simulink model "SimulinkModel"  (R2023b)
settings: Solver=VariableStepAuto  StartTime=0.0  StopTime=10.0  RelTol=1e-3
libraries: simulink x20, simulink_extras x7
settings Model: Creator=oykusucuoglu  LastModifiedBy=oykusucuoglu
settings OptimizationCC: ReuseModelBlockBuffer=off

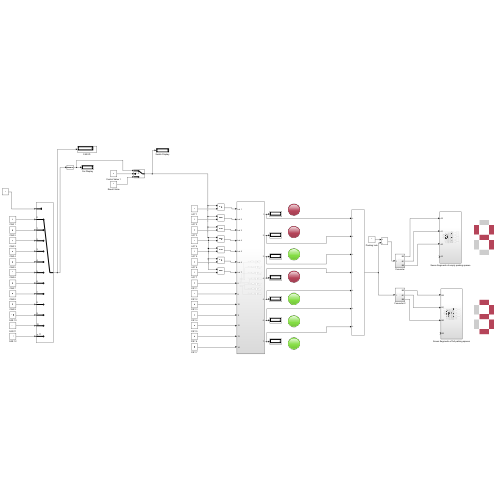
[thumbnail: Simulink's stored preview of the top-level diagram]
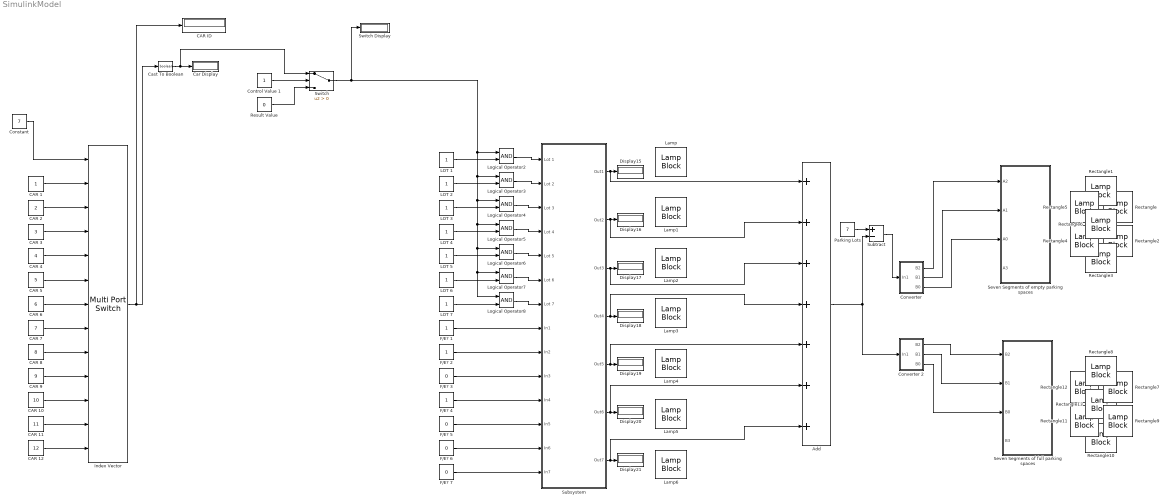
== system SimulinkModel ==
  Add : Sum  Inputs=+++++++
  CAR 1 : Constant
  CAR 10 : Constant  Value=10
  CAR 11 : Constant  Value=11
  CAR 12 : Constant  Value=12
  CAR 2 : Constant  Value=2
  CAR 3 : Constant  Value=3
  CAR 4 : Constant  Value=4
  CAR 5 : Constant  Value=5
  CAR 6 : Constant  Value=6
  CAR 7 : Constant  Value=7
  CAR 8 : Constant  Value=8
  CAR 9 : Constant  Value=9
  "CAR ID " : Display
  Car Display : Display
  Cast To Boolean : DataTypeConversion  OutDataTypeStr=boolean  SaturateOnIntegerOverflow=off  RndMeth=Floor
  Constant : Constant  Value=7
  Control Value 1 : Constant
  Converter : Subsystem
  Converter 2 : Subsystem
  Display{15..21} (7 alike) : Display
  F/E? 1 : Constant
  F/E? 2 : Constant
  F/E? 3 : Constant  Value=0
  F/E? 4 : Constant
  F/E? 5 : Constant  Value=0
  "F/E? 6 " : Constant  Value=0
  F/E? 7 : Constant  Value=0
  Index Vector : MultiPortSwitch  DataPortOrder=Zero-based contiguous  Inputs=12  zeroidx=on  SaturateOnIntegerOverflow=off  InputSameDT=off
  LOT {1..7} (7 alike) : Constant
  Lamp{,1..6} (7 alike) : LampBlock  LabelPosition=Hide
  Logical Operator{2..8} (7 alike) : Logic  AllPortsSameDT=off  OutDataTypeStr=boolean
  Parking Lots : Constant  Value=7
  Rectangle{,1..13} (14 alike) : LampBlock  LabelPosition=Hide  Icon=Rectangle
  Result Value : Constant  Value=0
  Seven Segments of empty parking spaces : Subsystem
  Seven Segments of full parking spaces : Subsystem
  Subsystem : Subsystem
  Subtract : Sum  Inputs=+-
  Switch : Switch  Criteria=u2 > Threshold  SaturateOnIntegerOverflow=off  InputSameDT=off
  Switch Display : Display
  wires:
  CAR 5/1 -> Index Vector/6
  CAR 11/1 -> Index Vector/12
  CAR 3/1 -> Index Vector/4
  CAR 2/1 -> Index Vector/3
  CAR 7/1 -> Index Vector/8
  CAR 10/1 -> Index Vector/11
  CAR 1/1 -> Index Vector/2
  Index Vector/1 -> "CAR ID "/1, Cast To Boolean/1
  CAR 4/1 -> Index Vector/5
  CAR 8/1 -> Index Vector/9
  CAR 6/1 -> Index Vector/7
  Constant/1 -> Index Vector/1
  CAR 12/1 -> Index Vector/13
  CAR 9/1 -> Index Vector/10
  Add/1 -> Converter 2/1(In1), Subtract/2
  Result Value/1 -> Switch/3
  Control Value 1/1 -> Switch/2
  Subsystem/2(Out2) -> Add/2, Display16/1
  Subsystem/3(Out3) -> Add/3, Display17/1
  Subsystem/4(Out4) -> Add/4, Display18/1
  Subsystem/5(Out5) -> Add/5, Display19/1
  Subsystem/6(Out6) -> Add/6, Display20/1
  Subsystem/7(Out7) -> Add/7, Display21/1
  Subsystem/1(Out1) -> Add/1, Display15/1
  Cast To Boolean/1 -> Switch/1, Car Display/1
  Parking Lots/1 -> Subtract/1
  "F/E? 6 "/1 -> Subsystem/13(In6)
  F/E? 4/1 -> Subsystem/11(In4)
  F/E? 7/1 -> Subsystem/14(In7)
  F/E? 1/1 -> Subsystem/8(In1)
  F/E? 5/1 -> Subsystem/12(In5)
  F/E? 3/1 -> Subsystem/10(In3)
  F/E? 2/1 -> Subsystem/9(In2)
  LOT 1/1 -> Logical Operator2/2
  LOT 2/1 -> Logical Operator3/2
  LOT 3/1 -> Logical Operator4/2
  Switch/1 -> Logical Operator8/1, Logical Operator7/1, Logical Operator6/1, Logical Operator5/1, Logical Operator4/1, Logical Operator3/1, Logical Operator2/1, Switch Display/1
  LOT 4/1 -> Logical Operator5/2
  LOT 5/1 -> Logical Operator6/2
  LOT 6/1 -> Logical Operator7/2
  LOT 7/1 -> Logical Operator8/2
  Logical Operator2/1 -> Subsystem/1(Lot 1)
  Logical Operator3/1 -> Subsystem/2(Lot 2)
  Logical Operator4/1 -> Subsystem/3(Lot 3)
  Logical Operator5/1 -> Subsystem/4(Lot 4)
  Logical Operator6/1 -> Subsystem/5(Lot 5)
  Logical Operator7/1 -> Subsystem/6(Lot 6)
  Logical Operator8/1 -> Subsystem/7(Lot 7)
  Subtract/1 -> Converter/1(In1)
  Converter/1(B2) -> Seven Segments of empty parking spaces/1(A2)
  Converter/2(B1) -> Seven Segments of empty parking spaces/2(A1)
  Converter/3(B0) -> Seven Segments of empty parking spaces/3(A0)
  Converter 2/1(B2) -> Seven Segments of full parking spaces/1(B2)
  Converter 2/2(B1) -> Seven Segments of full parking spaces/2(B1)
  Converter 2/3(B0) -> Seven Segments of full parking spaces/3(B0)

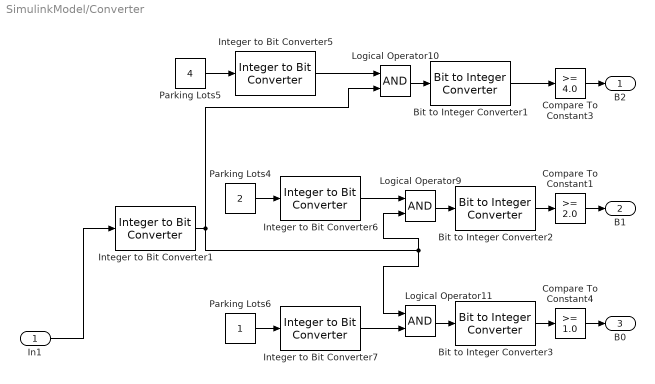
== system SimulinkModel/Converter ==
  In1 : Inport
  Bit to Integer Converter1 : simulink/Logic and Bit Operations/Bit to Integer Converter  nbits=3  bitOrder=MSB first  signedOutputValues=Unsigned  outDtype=Inherit via internal rule  outDtypeSigned=Inherit via internal rule
  Bit to Integer Converter2 : simulink/Logic and Bit Operations/Bit to Integer Converter  nbits=3  bitOrder=MSB first  signedOutputValues=Unsigned  outDtype=Inherit via internal rule  outDtypeSigned=Inherit via internal rule
  Bit to Integer Converter3 : simulink/Logic and Bit Operations/Bit to Integer Converter  nbits=3  bitOrder=MSB first  signedOutputValues=Unsigned  outDtype=Inherit via internal rule  outDtypeSigned=Inherit via internal rule
  Compare To Constant1 : simulink/Logic and Bit Operations/Compare To Constant  relop=>=  const=2.0  OutDataTypeStr=boolean
  Compare To Constant3 : simulink/Logic and Bit Operations/Compare To Constant  relop=>=  const=4.0  OutDataTypeStr=boolean
  Compare To Constant4 : simulink/Logic and Bit Operations/Compare To Constant  relop=>=  const=1.0  OutDataTypeStr=boolean
  Integer to Bit Converter{1,5..7} (4 alike) : simulink/Logic and Bit Operations/Integer to Bit Converter  nbits=3  signedInputValues=Unsigned  bitOrder=MSB first  outDtype=Inherit via internal rule
  Logical Operator10 : Logic  AllPortsSameDT=off  OutDataTypeStr=boolean
  Logical Operator11 : Logic  AllPortsSameDT=off  OutDataTypeStr=boolean
  Logical Operator9 : Logic  AllPortsSameDT=off  OutDataTypeStr=boolean
  Parking Lots4 : Constant  Value=2
  Parking Lots5 : Constant  Value=4
  Parking Lots6 : Constant
  B2 : Outport
  B1 : Outport  Port=2
  B0 : Outport  Port=3
  wires:
  Bit to Integer Converter2/1 -> Compare To Constant1/1
  Integer to Bit Converter1/1 -> Logical Operator10/2, Logical Operator11/1, Logical Operator9/2
  Parking Lots5/1 -> Integer to Bit Converter5/1
  Logical Operator9/1 -> Bit to Integer Converter2/1
  Logical Operator10/1 -> Bit to Integer Converter1/1
  Bit to Integer Converter1/1 -> Compare To Constant3/1
  Integer to Bit Converter7/1 -> Logical Operator11/2
  Integer to Bit Converter5/1 -> Logical Operator10/1
  Parking Lots4/1 -> Integer to Bit Converter6/1
  In1/1 -> Integer to Bit Converter1/1
  Integer to Bit Converter6/1 -> Logical Operator9/1
  Logical Operator11/1 -> Bit to Integer Converter3/1
  Parking Lots6/1 -> Integer to Bit Converter7/1
  Bit to Integer Converter3/1 -> Compare To Constant4/1
  Compare To Constant4/1 -> B0/1
  Compare To Constant1/1 -> B1/1
  Compare To Constant3/1 -> B2/1

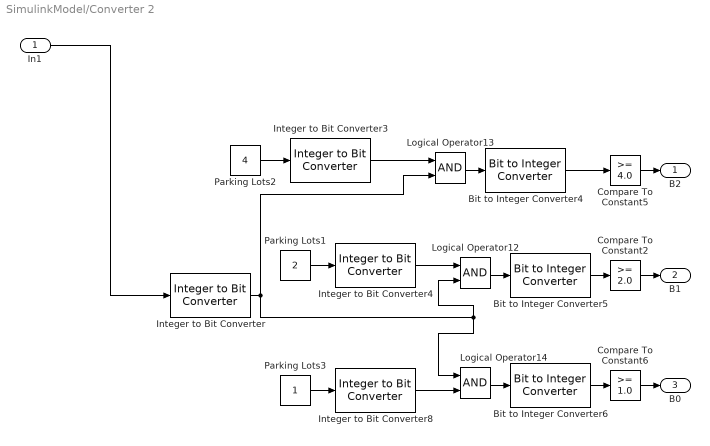
== system SimulinkModel/Converter 2 ==
  In1 : Inport
  Bit to Integer Converter4 : simulink/Logic and Bit Operations/Bit to Integer Converter  nbits=3  bitOrder=MSB first  signedOutputValues=Unsigned  outDtype=Inherit via internal rule  outDtypeSigned=Inherit via internal rule
  Bit to Integer Converter5 : simulink/Logic and Bit Operations/Bit to Integer Converter  nbits=3  bitOrder=MSB first  signedOutputValues=Unsigned  outDtype=Inherit via internal rule  outDtypeSigned=Inherit via internal rule
  Bit to Integer Converter6 : simulink/Logic and Bit Operations/Bit to Integer Converter  nbits=3  bitOrder=MSB first  signedOutputValues=Unsigned  outDtype=Inherit via internal rule  outDtypeSigned=Inherit via internal rule
  Compare To Constant2 : simulink/Logic and Bit Operations/Compare To Constant  relop=>=  const=2.0  OutDataTypeStr=boolean
  Compare To Constant5 : simulink/Logic and Bit Operations/Compare To Constant  relop=>=  const=4.0  OutDataTypeStr=boolean
  Compare To Constant6 : simulink/Logic and Bit Operations/Compare To Constant  relop=>=  const=1.0  OutDataTypeStr=boolean
  Integer to Bit Converter{,3..4,8} (4 alike) : simulink/Logic and Bit Operations/Integer to Bit Converter  nbits=3  signedInputValues=Unsigned  bitOrder=MSB first  outDtype=Inherit via internal rule
  Logical Operator12 : Logic  AllPortsSameDT=off  OutDataTypeStr=boolean
  Logical Operator13 : Logic  AllPortsSameDT=off  OutDataTypeStr=boolean
  Logical Operator14 : Logic  AllPortsSameDT=off  OutDataTypeStr=boolean
  Parking Lots1 : Constant  Value=2
  Parking Lots2 : Constant  Value=4
  Parking Lots3 : Constant
  B2 : Outport
  B1 : Outport  Port=2
  B0 : Outport  Port=3
  wires:
  Compare To Constant2/1 -> B1/1
  Logical Operator12/1 -> Bit to Integer Converter5/1
  Parking Lots2/1 -> Integer to Bit Converter3/1
  Integer to Bit Converter/1 -> Logical Operator13/2, Logical Operator14/1, Logical Operator12/2
  Parking Lots1/1 -> Integer to Bit Converter4/1
  Compare To Constant5/1 -> B2/1
  Logical Operator13/1 -> Bit to Integer Converter4/1
  Bit to Integer Converter4/1 -> Compare To Constant5/1
  Bit to Integer Converter5/1 -> Compare To Constant2/1
  Integer to Bit Converter3/1 -> Logical Operator13/1
  Bit to Integer Converter6/1 -> Compare To Constant6/1
  Logical Operator14/1 -> Bit to Integer Converter6/1
  Integer to Bit Converter8/1 -> Logical Operator14/2
  Integer to Bit Converter4/1 -> Logical Operator12/1
  Parking Lots3/1 -> Integer to Bit Converter8/1
  In1/1 -> Integer to Bit Converter/1
  Compare To Constant6/1 -> B0/1

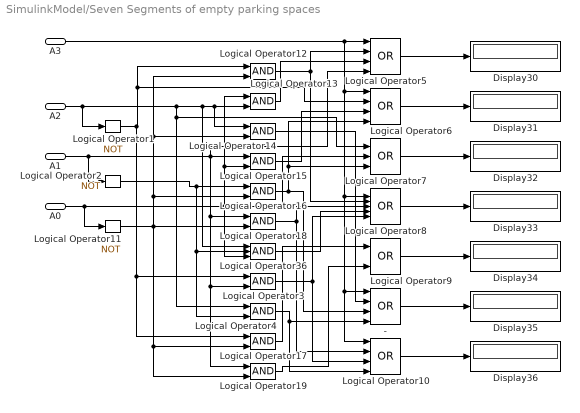
== system SimulinkModel/Seven Segments of empty parking spaces ==
  A2 : Inport
  A1 : Inport  Port=2
  A0 : Inport  Port=3
  A3 : Inport  Port=4
  "   -" : Logic  Operator=OR  Inputs=4  AllPortsSameDT=off  OutDataTypeStr=boolean
  Display{30..36} (7 alike) : Display
  Logical Operator1 : Logic  Operator=NOT  AllPortsSameDT=off  OutDataTypeStr=boolean
  Logical Operator10 : Logic  Operator=OR  Inputs=4  AllPortsSameDT=off  OutDataTypeStr=boolean
  Logical Operator11 : Logic  Operator=NOT  AllPortsSameDT=off  OutDataTypeStr=boolean
  Logical Operator{3..4,12..19} (10 alike) : Logic  AllPortsSameDT=off  OutDataTypeStr=boolean
  Logical Operator2 : Logic  Operator=NOT  AllPortsSameDT=off  OutDataTypeStr=boolean
  Logical Operator36 : Logic  Inputs=3  AllPortsSameDT=off  OutDataTypeStr=boolean
  Logical Operator5 : Logic  Operator=OR  Inputs=4  AllPortsSameDT=off  OutDataTypeStr=boolean
  Logical Operator6 : Logic  Operator=OR  Inputs=4  AllPortsSameDT=off  OutDataTypeStr=boolean
  Logical Operator7 : Logic  Operator=OR  Inputs=3  AllPortsSameDT=off  OutDataTypeStr=boolean
  Logical Operator8 : Logic  Operator=OR  Inputs=5  AllPortsSameDT=off  OutDataTypeStr=boolean
  Logical Operator9 : Logic  Operator=OR  AllPortsSameDT=off  OutDataTypeStr=boolean
  wires:
  Logical Operator9/1 -> Display34/1
  Logical Operator8/1 -> Display33/1
  Logical Operator7/1 -> Display32/1
  Logical Operator14/1 -> "   -"/2
  Logical Operator6/1 -> Display31/1
  Logical Operator10/1 -> Display36/1
  Logical Operator1/1 -> Logical Operator17/1, Logical Operator3/1, Logical Operator6/2, Logical Operator12/1
  Logical Operator11/1 -> Logical Operator19/2, Logical Operator17/2, Logical Operator18/2, Logical Operator16/2, Logical Operator14/2, Logical Operator12/2
  Logical Operator3/1 -> Logical Operator10/3, Logical Operator8/5
  Logical Operator15/1 -> Logical Operator6/3
  Logical Operator4/1 -> Logical Operator10/4, "   -"/4
  A2/1 -> Logical Operator7/1, Logical Operator4/1, Logical Operator36/1, Logical Operator14/1, Logical Operator13/2, Logical Operator1/1
  A1/1 -> Logical Operator19/1, Logical Operator3/2, Logical Operator18/1, Logical Operator5/4, Logical Operator15/1, Logical Operator2/1
  Logical Operator5/1 -> Display30/1
  A0/1 -> Logical Operator11/1, Logical Operator36/3, Logical Operator7/2, Logical Operator15/2, Logical Operator13/1
  "   -"/1 -> Display35/1
  Logical Operator13/1 -> Logical Operator5/3
  Logical Operator12/1 -> Logical Operator8/2, Logical Operator5/2
  Logical Operator2/1 -> Logical Operator4/2, Logical Operator36/2, Logical Operator16/1
  Logical Operator18/1 -> Logical Operator10/2, Logical Operator8/3
  Logical Operator36/1 -> Logical Operator8/4
  Logical Operator16/1 -> "   -"/3, Logical Operator7/3, Logical Operator6/4
  A3/1 -> Logical Operator10/1, "   -"/1, Logical Operator8/1, Logical Operator6/1, Logical Operator5/1
  Logical Operator17/1 -> Logical Operator9/1
  Logical Operator19/1 -> Logical Operator9/2

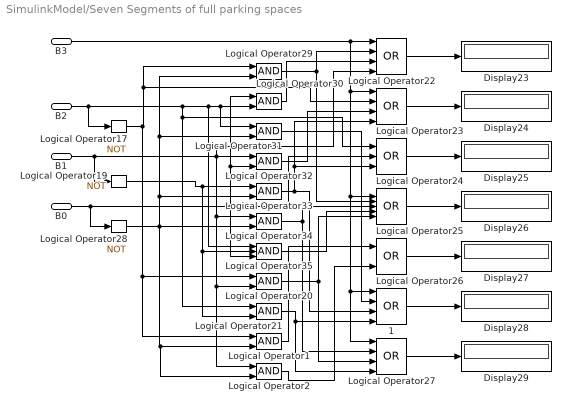
== system SimulinkModel/Seven Segments of full parking spaces ==
  B2 : Inport
  B1 : Inport  Port=2
  B0 : Inport  Port=3
  B3 : Inport  Port=4
  "   1" : Logic  Operator=OR  Inputs=4  AllPortsSameDT=off  OutDataTypeStr=boolean
  Display{23..29} (7 alike) : Display
  Logical Operator{1..2,20..21,29..34} (10 alike) : Logic  AllPortsSameDT=off  OutDataTypeStr=boolean
  Logical Operator17 : Logic  Operator=NOT  AllPortsSameDT=off  OutDataTypeStr=boolean
  Logical Operator19 : Logic  Operator=NOT  AllPortsSameDT=off  OutDataTypeStr=boolean
  Logical Operator22 : Logic  Operator=OR  Inputs=4  AllPortsSameDT=off  OutDataTypeStr=boolean
  Logical Operator23 : Logic  Operator=OR  Inputs=4  AllPortsSameDT=off  OutDataTypeStr=boolean
  Logical Operator24 : Logic  Operator=OR  Inputs=3  AllPortsSameDT=off  OutDataTypeStr=boolean
  Logical Operator25 : Logic  Operator=OR  Inputs=5  AllPortsSameDT=off  OutDataTypeStr=boolean
  Logical Operator26 : Logic  Operator=OR  AllPortsSameDT=off  OutDataTypeStr=boolean
  Logical Operator27 : Logic  Operator=OR  Inputs=4  AllPortsSameDT=off  OutDataTypeStr=boolean
  Logical Operator28 : Logic  Operator=NOT  AllPortsSameDT=off  OutDataTypeStr=boolean
  Logical Operator35 : Logic  Inputs=3  AllPortsSameDT=off  OutDataTypeStr=boolean
  wires:
  Logical Operator26/1 -> Display27/1
  Logical Operator23/1 -> Display24/1
  Logical Operator22/1 -> Display23/1
  Logical Operator27/1 -> Display29/1
  Logical Operator35/1 -> Logical Operator25/4
  Logical Operator32/1 -> Logical Operator23/3
  "   1"/1 -> Display28/1
  Logical Operator24/1 -> Display25/1
  Logical Operator30/1 -> Logical Operator22/3
  Logical Operator28/1 -> Logical Operator2/2, Logical Operator1/2, Logical Operator34/2, Logical Operator33/2, Logical Operator31/2, Logical Operator29/2
  Logical Operator17/1 -> Logical Operator1/1, Logical Operator20/1, Logical Operator23/2, Logical Operator29/1
  B3/1 -> Logical Operator27/1, "   1"/1, Logical Operator25/1, Logical Operator23/1, Logical Operator22/1
  B1/1 -> Logical Operator22/4, Logical Operator2/1, Logical Operator20/2, Logical Operator34/1, Logical Operator32/1, Logical Operator19/1
  B0/1 -> Logical Operator28/1, Logical Operator35/3, Logical Operator24/2, Logical Operator32/2, Logical Operator30/1
  Logical Operator20/1 -> Logical Operator27/3, Logical Operator25/5
  Logical Operator21/1 -> Logical Operator27/4, "   1"/4
  Logical Operator33/1 -> "   1"/3, Logical Operator24/3, Logical Operator23/4
  Logical Operator25/1 -> Display26/1
  Logical Operator31/1 -> "   1"/2
  Logical Operator34/1 -> Logical Operator27/2, Logical Operator25/3
  B2/1 -> Logical Operator24/1, Logical Operator21/1, Logical Operator35/1, Logical Operator31/1, Logical Operator30/2, Logical Operator17/1
  Logical Operator19/1 -> Logical Operator21/2, Logical Operator35/2, Logical Operator33/1
  Logical Operator29/1 -> Logical Operator25/2, Logical Operator22/2
  Logical Operator1/1 -> Logical Operator26/1
  Logical Operator2/1 -> Logical Operator26/2

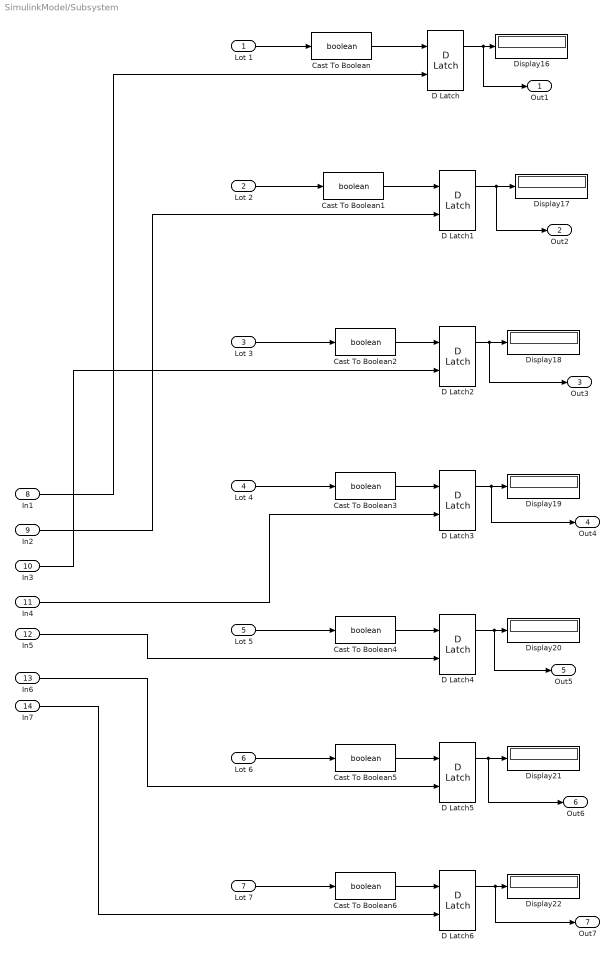
== system SimulinkModel/Subsystem ==
  Lot 1 : Inport
  Lot 2 : Inport  Port=2
  Lot 3 : Inport  Port=3
  Lot 4 : Inport  Port=4
  Lot 5 : Inport  Port=5
  Lot 6 : Inport  Port=6
  Lot 7 : Inport  Port=7
  In1 : Inport  Port=8
  In2 : Inport  Port=9
  In3 : Inport  Port=10
  In4 : Inport  Port=11
  In5 : Inport  Port=12
  In6 : Inport  Port=13
  In7 : Inport  Port=14
  Cast To Boolean{,1..6} (7 alike) : DataTypeConversion  OutDataTypeStr=boolean  SaturateOnIntegerOverflow=off  RndMeth=Floor
  D Latch{,1..6} (7 alike) : simulink_extras/Flip Flops/D Latch
  Display{16..22} (7 alike) : Display
  Out1 : Outport
  Out2 : Outport  Port=2
  Out3 : Outport  Port=3
  Out4 : Outport  Port=4
  Out5 : Outport  Port=5
  Out6 : Outport  Port=6
  Out7 : Outport  Port=7
  wires:
  D Latch/1 -> Out1/1, Display16/1
  Cast To Boolean/1 -> D Latch/1
  Lot 1/1 -> Cast To Boolean/1
  Lot 2/1 -> Cast To Boolean1/1
  Cast To Boolean1/1 -> D Latch1/1
  Lot 3/1 -> Cast To Boolean2/1
  Cast To Boolean2/1 -> D Latch2/1
  Cast To Boolean3/1 -> D Latch3/1
  Lot 4/1 -> Cast To Boolean3/1
  Cast To Boolean4/1 -> D Latch4/1
  Lot 5/1 -> Cast To Boolean4/1
  Cast To Boolean5/1 -> D Latch5/1
  Lot 6/1 -> Cast To Boolean5/1
  Cast To Boolean6/1 -> D Latch6/1
  Lot 7/1 -> Cast To Boolean6/1
  D Latch1/1 -> Out2/1, Display17/1
  D Latch3/1 -> Out4/1, Display19/1
  D Latch4/1 -> Out5/1, Display20/1
  D Latch5/1 -> Out6/1, Display21/1
  D Latch6/1 -> Out7/1, Display22/1
  In1/1 -> D Latch/2
  In2/1 -> D Latch1/2
  In3/1 -> D Latch2/2
  In4/1 -> D Latch3/2
  In5/1 -> D Latch4/2
  In6/1 -> D Latch5/2
  In7/1 -> D Latch6/2
  D Latch2/1 -> Out3/1, Display18/1
